simulink model "PlantOnlyTest"  (R2014a)
settings: Solver=ode45  StartTime=0.0  StopTime=5  RelTol=1e-3
values from neighbouring files (symbols this model uses):
  K_PWM = PWM_res/V_rail    (= 83.3333333333)    [ControlDesign.m]    (also in ControlDesignForceModeLinear.m = 0.012)
  PulsePeakAmplitude = 5    [ControlDesign.m]
  PWM_res = 2000    [ControlDesign.m]    (also in ControlDesignForceModeLinear.m)
settings Model: Creator=oberstare  LastModifiedBy=oberstare

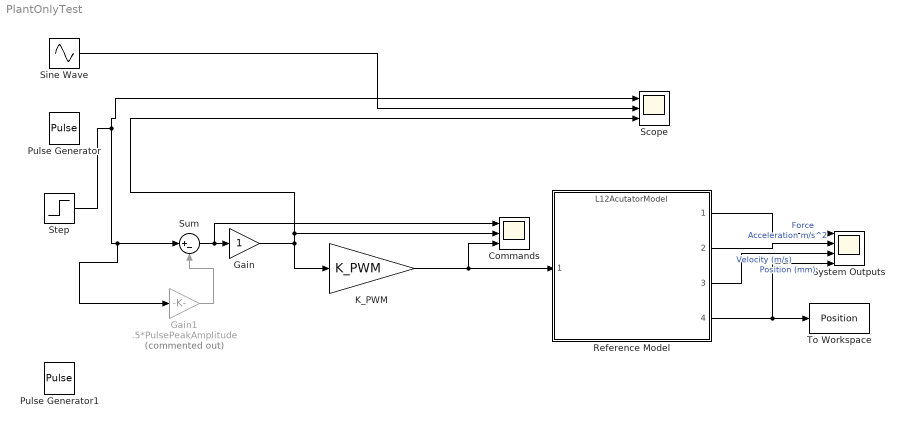
== system PlantOnlyTest ==
  Commands : Scope  NumInputPorts=3
      settings: YMin=0~0~0  YMax=5~5~450
  Gain : Gain
  Gain1 : Gain  Commented=on  Gain=.5*PulsePeakAmplitude
  K_PWM : Gain  Gain=K_PWM
  Pulse Generator : DiscretePulseGenerator  PulseType=Time based  Amplitude=PulsePeakAmplitude  Period=1  PhaseDelay=.2
  Pulse Generator1 : DiscretePulseGenerator  Period=1000
  Reference Model : ModelReference  ModelNameDialog=L12AcutatorModel.slx  SimulationMode=Normal  ModelReferenceVersion=1.40  CopyOfModelName=L12AcutatorModel.slx  DefaultDataLogging=on
  Scope : Scope  NumInputPorts=3
      settings: YMin=0~2199.96~-1  YMax=5~2200~1  SaveName=ScopeData7
  Sine Wave : Sin  Amplitude=PWM_res/10  Bias=PWM_res  Frequency=.1  Phase=pi/2  SampleTime=0
  Step : Step  After=1.5  SampleTime=0
  Sum : Sum  Inputs=|+-
  System Outputs : Scope  NumInputPorts=4
      settings: YMin=0~0~0~0  YMax=0.013~0.175~0.005~0.375
  To Workspace : ToWorkspace  VariableName=Position  SaveFormat=Timeseries  SampleTime=-1
  wires:
  Gain/1 -> K_PWM/1, Commands/2, Scope/3
  Gain1/1 -> Sum/2
  Sum/1 -> Commands/1, Gain/1
  Sine Wave/1 -> Scope/2
  Reference Model/1 -> System Outputs/1  "Force"
  Reference Model/2 -> System Outputs/2  "Acceleration m/s^2"
  Reference Model/4 -> To Workspace/1, System Outputs/4  "Position (mm)"
  Reference Model/3 -> System Outputs/3  "Velocity (m/s)"
  K_PWM/1 -> Commands/3, Reference Model/1
  Step/1 -> Scope/1, Gain1/1, Sum/1
